simulink model "Simulink_demo_2024"  (R2024a)
settings: Solver=ode4  StartTime=0.0  StopTime=200  FixedStep=1e-3  RelTol=1e-3
settings Model: Creator=20225074  LastModifiedBy=20231620
settings DebuggingCC: UnderSpecifiedDimensionMsg=warning

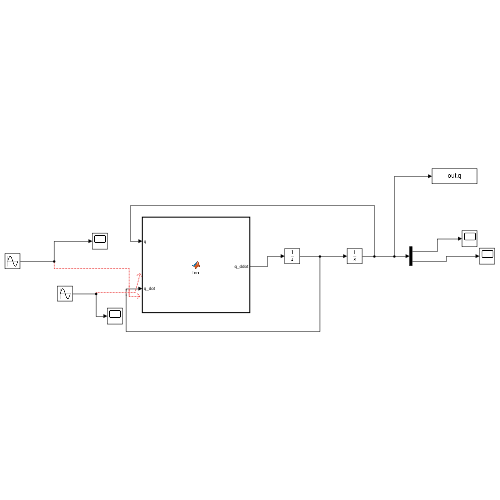
[thumbnail: Simulink's stored preview of the top-level diagram]
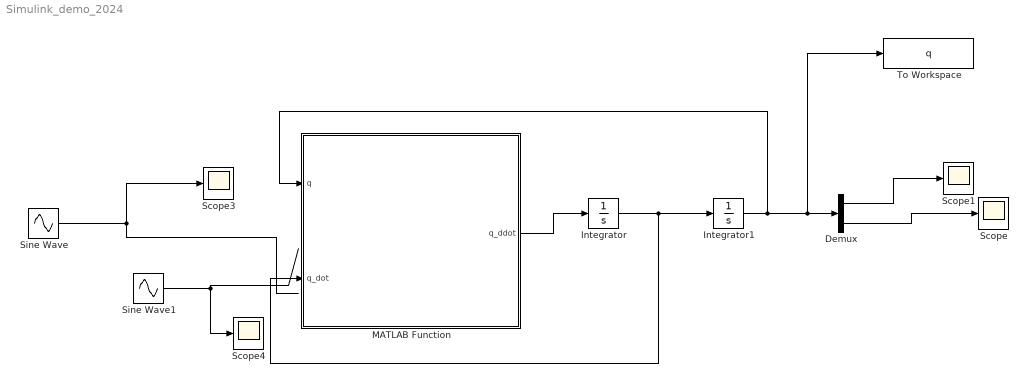
== system Simulink_demo_2024 ==
  Demux : Demux  Outputs=2
  Integrator : Integrator  InitialCondition=[0;0]
  Integrator1 : Integrator  InitialCondition=[1.1;1.7]
  MATLAB Function : MATLAB Function  TreatAsAtomicUnit=on
  Scope{,1,3..4} (4 alike) : Scope
  Sine Wave : Sin  Amplitude=-4/5  Frequency=2  SampleTime=0
  Sine Wave1 : Sin  Amplitude=1/2  SampleTime=0
  To Workspace : ToWorkspace  VariableName=q  SampleTime=-1
  wires:
  MATLAB Function/1(q_ddot) -> Integrator/1
  Integrator/1 -> MATLAB Function/2(q_dot), Integrator1/1
  Integrator1/1 -> To Workspace/1, Demux/1, MATLAB Function/1(q)
  Sine Wave/1 -> Scope3/1
  Demux/1 -> Scope1/1
  Demux/2 -> Scope/1
  Sine Wave1/1 -> Scope4/1

== matlab function Simulink_demo_2024/MATLAB Function ==
  data: q input; q_ddot output; q_dot input

function q_ddot = fcn(q, q_dot)

% System parameters
g = 9.81;
l_p = 0.5;
l_w = 1;
m_p = 1;
m_w = 0.2;
r_w = 0.2;
J_p = 0.083;
J_w = 0.1;
d_phi = 0.2;
k_theta = 6.558;
d_theta = 0.1;
theta_ref = pi/2;
k_phi = 0.114;
phi_ref = pi/2;
tau = 0;
theta = q(1);
phi = q(2);
theta_dot = q_dot(1);
phi_dot = q_dot(2);

x = 0;
x_dot = 0;
x_ddot = 0;

M = [2*m_p*l_p^2 + 2*m_w*l_w^2 + 2*J_p + 2*J_w, 2*J_w; J_w, J_w];

F = [0; 0];

F(1) = -2*d_theta*theta_dot - k_theta*(2*theta - 2*theta_ref) - 2*g*l_p*m_p*cos(theta) - 2*g*l_w*m_w*cos(theta) - 2*theta_dot*x_dot*cos(theta)*(l_p*m_p + l_w*m_w) + (x_ddot*sin(theta) + theta_dot*x_dot*cos(theta))*(2*l_p*m_p + 2*l_w*m_w);

F(2) = tau - k_phi*(phi - phi_ref) - d_phi*phi_dot;

q_ddot = M\F;
